simulink model "UR5_SAC_Sim"  (R2022a)
settings: Solver=FixedStepDiscrete  StartTime=0.0  StopTime=Nmax*Ts  FixedStep=Ts  RelTol=1e-3
model workspace (MAT data in the model file):
  AngularProgressWeight = 10
  BaseTransform = [0  -1  0  0; 1  0  0  0; 0  0  1  0; 0  0  0  1]
  FixedTransforms = reshape([1 0 0 0 0 1 0 0 0 0 1 0 0 0 0.163 1 0 0 -1 0 0 1 0 0 1 0 0 0 0 0.138 0 1 1 0 0 0 0 1 0 0 0 0 1 0 0 -0.131 0.425 1 0 0 -1 0 0 1 0 0 1 0 0 0 0 0 0.392 1 1 0 0 0 0 1 0 0 0 0 1 0 0 0.127 0 1 1 0 0 0 0 1 0 0 0 0 1 0 0 0 0.1 1], [4 4 6])
  GeometryID = 'Lec05_UR5e_7352274f6c21'
  InitialEa = 0.349065850399
  InitialEd = 1.12690565409
  JointAxes = [0  0  0  0  0  0; 0  1  1  1  0  1; 1  0  0  0  1  0]
  Nmax = 200
  ObsScale = [0.159154943092; 0.159154943092; 0.159154943092; 0.159154943092; 0.159154943092; 0.159154943092; 1; 1; 1; 1; 1; 1; 1; 1; 1]
  ProgressWeight = 100
  SuccessBonus = 50
  ToolTransform = [0  1  0  0; 0  0  1  0.1; 1  0  0  0; 0  0  0  1]
  Ts = 0.05
  dqMax = [0.0349065850399; 0.0349065850399; 0.0349065850399; 0.0349065850399; 0.0349065850399; 0.0349065850399]
  eps_a = 0.0174532925199
  eps_d = 0.005
  pg = [-0.170034382667; -0.630912218479; 0.40033001611]
  q0 = [0; -1.57079632679; 1.57079632679; -1.57079632679; -1.57079632679; 0]
  qGoal = [2.61799387799; -1.2217304764; 1.3962634016; -1.74532925199; -1.2217304764; 0.349065850399]
  qMax = [6.28319; 6.28319; 3.1415; 6.28319; 6.28319; 6.28319]
  qMin = [-6.28319; -6.28319; -3.1415; -6.28319; -6.28319; -6.28319]
  vg = [0.296198132726; -0.171010071663; -0.939692620786]
  wa = 10
  wd = 10
libraries: rllib x1
settings Model: Creator=admin  LastModifiedBy=admin

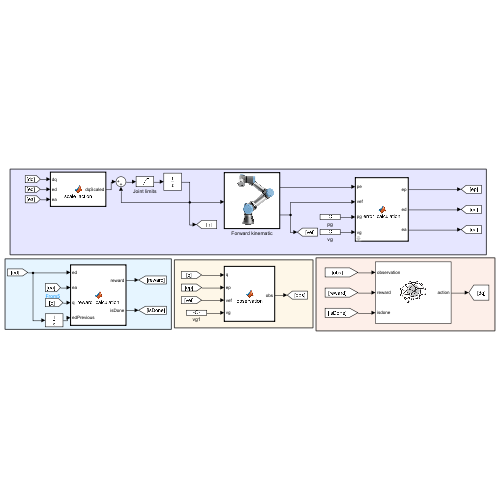
[thumbnail: Simulink's stored preview of the top-level diagram]
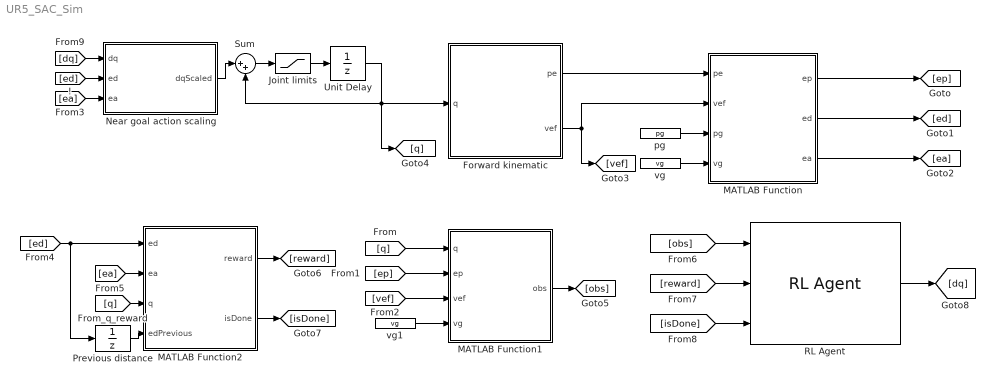
== system UR5_SAC_Sim ==
  Forward kinematic : MATLAB Function  TreatAsAtomicUnit=on
  Joint limits : Saturate  UpperLimit=qMax  LowerLimit=qMin
  MATLAB Function : MATLAB Function  TreatAsAtomicUnit=on
  MATLAB Function1 : MATLAB Function  TreatAsAtomicUnit=on
  MATLAB Function2 : MATLAB Function  TreatAsAtomicUnit=on
  Near goal action scaling : MATLAB Function  TreatAsAtomicUnit=on
  Previous distance : UnitDelay  InitialCondition=InitialEd  SampleTime=Ts  HasFrameUpgradeWarning=on
  RL Agent : rllib/RL Agent  Agent=agent  ExternalActionAsInput=off  ProvideLastAction=off  ProvideCumRwd=off  TreatAsDirectFeedthrough=on  UseStrictObservationDataTypes=off
  Sum : Sum  Inputs=|++
  Unit Delay : UnitDelay  InitialCondition=q0  SampleTime=Ts  HasFrameUpgradeWarning=on
  pg : Constant  Value=pg
  vg : Constant  Value=vg
  vg1 : Constant  Value=vg
  wires:
  Unit Delay/1 -> Forward kinematic/1(q), Sum/2, [q]
  Forward kinematic/1(pe) -> MATLAB Function/1(pe)
  Forward kinematic/2(vef) -> [vef], MATLAB Function/2(vef)
  MATLAB Function/1(ep) -> [ep]
  MATLAB Function/2(ed) -> [ed]
  MATLAB Function/3(ea) -> [ea]
  [q] -> MATLAB Function1/1(q)
  [ep] -> MATLAB Function1/2(ep)
  [vef] -> MATLAB Function1/3(vef)
  MATLAB Function1/1(obs) -> [obs]
  [ed] -> MATLAB Function2/1(ed), Previous distance/1
  [ea] -> MATLAB Function2/2(ea)
  MATLAB Function2/1(reward) -> [reward]
  MATLAB Function2/2(isDone) -> [isDone]
  [obs] -> RL Agent/1
  [reward] -> RL Agent/2
  [isDone] -> RL Agent/3
  RL Agent/1 -> [dq]
  vg/1 -> MATLAB Function/4(vg)
  pg/1 -> MATLAB Function/3(pg)
  Sum/1 -> Joint limits/1
  Joint limits/1 -> Unit Delay/1
  vg1/1 -> MATLAB Function1/4(vg)
  [q] -> MATLAB Function2/3(q)
  [dq] -> Near goal action scaling/1(dq)
  [ed] -> Near goal action scaling/2(ed)
  Near goal action scaling/1(dqScaled) -> Sum/1
  Previous distance/1 -> MATLAB Function2/4(edPrevious)
  [ea] -> Near goal action scaling/3(ea)

== matlab function UR5_SAC_Sim/MATLAB Function ==
  data: pe input; ep output; vef input; pg input; vg input; ed output; ea output
function [ep,ed,ea] = error_calculation(pe,vef,pg,vg)

ep = pg - pe;

ed = norm(ep);

c = dot(vef,vg);

c = min(1,max(-1,c));

ea = acos(c);

end

== matlab function UR5_SAC_Sim/Forward kinematic ==
  data: q input; pe output; vef output; BaseTransform parameter; FixedTransforms parameter; JointAxes parameter; ToolTransform parameter
function [pe,vef] = XML_FK(q, BaseTransform, FixedTransforms, JointAxes, ToolTransform)
%#codegen
% Exact chain from the user-provided Lec05 ur5e.xml.
% Parameters are saved in Model Workspace, not read from external M-files.
T=BaseTransform;
for i=1:6
    a=JointAxes(:,i); c=cos(q(i)); s=sin(q(i));
    K=[0,-a(3),a(2);a(3),0,-a(1);-a(2),a(1),0];
    J=eye(4); J(1:3,1:3)=c*eye(3)+(1-c)*(a*a')+s*K;
    T=T*FixedTransforms(:,:,i)*J;
end
T=T*ToolTransform;
pe=T(1:3,4); vef=T(1:3,3); vef=vef/norm(vef);
end

== matlab function UR5_SAC_Sim/MATLAB Function1 ==
  data: q input; obs output; ep input; vef input; vg input
function obs = observation(q,ep,vef,vg)
obs=[q/(2*pi);ep;vef;vg];
end

== matlab function UR5_SAC_Sim/MATLAB Function2 ==
  data: ed input; reward output; ea input; isDone output; q input; edPrevious input; qMin parameter; qMax parameter
function [reward,isDone] = reward_calculation(ed,ea,q,edPrevious,qMin,qMax)
% Tiered pose reward with explicit precision and stagnation signals.
distanceChange=abs(ed-edPrevious);
distanceProgress=edPrevious-ed;
qn=2*(q-(qMin+qMax)/2)./(qMax-qMin);
limitPenalty=sum(max(abs(qn)-0.85,0).^2);
success=(ed<=0.005)&&(ea<=0.017453292519943295);
if ed>0.05
    R0=-ed/1.12690565408916-2*ea/pi;
    reward=R0-1+100*distanceProgress-0.2*limitPenalty;
elseif ed>0.005
    R0=-ed/0.05-0.25*ea/0.017453292519943295;
    reward=R0+2+100*distanceProgress-0.2*limitPenalty;
else
    R0=-ed/0.005-0.25*ea/0.017453292519943295;
    reward=R0+4+100*distanceProgress-0.2*limitPenalty;
end
if ed<=0.005 && ea<=0.0872664625997165
    reward=reward+5;
end
if ~success && distanceChange<1e-4
    reward=reward-0.5;
end
if success
    reward=reward+25;
end
isDone=success;
end

== matlab function UR5_SAC_Sim/Near goal action scaling ==
  data: dq input; dqScaled output; ed input; ea input
function dqScaled = scale_action(dq,ed,ea)
% Slow down only when both position and orientation errors are small.
combinedError=max(ed/0.03,ea/0.174532925199433);
alpha=max(0.05,min(1,combinedError));
dqScaled=alpha*dq;
end
